simulink model "modelo_LTI_equivalente_dinamica_residual"  (R2020a)
settings: Solver=VariableStepAuto  StartTime=0.0  StopTime=10.0  RelTol=1e-3
model workspace: external: MATLAB File D:\Ferran\Facultad\UNCuyo\Meca\Automática y Máquinas Eléctricas\Proyecto final\matlab2\parametros_y_especs\parametros_y_especif.m (data not in the file)
undefined symbols (not defined in the file): beq, Cts, Jeq, lambda_m, Ld, Lq, magnitude, Pp, r, Rs, Rts_amb
settings Model: Creator=Ferran  LastModifiedBy=Ferran

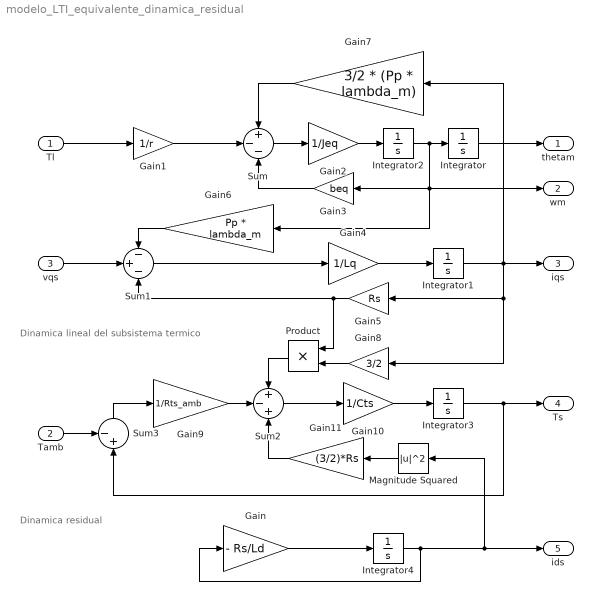
== system modelo_LTI_equivalente_dinamica_residual ==
  note: Dinamica residual
  note: Dinamica lineal del
      |  subsistema termico
  Tl : Inport
  Tamb : Inport  Port=2
  vqs : Inport  Port=3
  Gain : Gain  Gain=- Rs/Ld
  Gain1 : Gain  Gain=1/r
  Gain10 : Gain  Gain=1/Cts
  Gain11 : Gain  Gain=(3/2)*Rs
  Gain2 : Gain  Gain=1/Jeq
  Gain3 : Gain  Gain=beq
  Gain4 : Gain  Gain=1/Lq
  Gain5 : Gain  Gain=Rs
  Gain6 : Gain  Gain=Pp * lambda_m
  Gain7 : Gain  Gain=3/2 * (Pp * lambda_m)
  Gain8 : Gain  Gain=3/2
  Gain9 : Gain  Gain=1/Rts_amb
  Integrator{,1..4} (5 alike) : Integrator
  Magnitude Squared : Math  Operator=magnitude^2  SaturateOnIntegerOverflow=on
  Product : Product
  Sum : Sum  Inputs=+--
  Sum1 : Sum  Inputs=-+-
  Sum2 : Sum  Inputs=+-+
  Sum3 : Sum  Inputs=-+|
  thetam : Outport
  wm : Outport  Port=2
  iqs : Outport  Port=3
  Ts : Outport  Port=4
  ids : Outport  Port=5
  wires:
  Integrator/1 -> thetam/1
  Integrator2/1 -> Integrator/1, Gain6/1, wm/1, Gain3/1
  Gain2/1 -> Integrator2/1
  Tl/1 -> Gain1/1
  Gain1/1 -> Sum/2
  Gain3/1 -> Sum/3
  Sum/1 -> Gain2/1
  Sum1/1 -> Gain4/1
  Gain4/1 -> Integrator1/1
  Integrator1/1 -> Gain8/1, Gain5/1, Gain7/1, iqs/1
  Gain5/1 -> Product/1, Sum1/3
  vqs/1 -> Sum1/2
  Gain6/1 -> Sum1/1
  Gain7/1 -> Sum/1
  Gain8/1 -> Product/2
  Product/1 -> Sum2/1
  Tamb/1 -> Sum3/1
  Sum3/1 -> Gain9/1
  Gain9/1 -> Sum2/2
  Sum2/1 -> Gain10/1
  Gain10/1 -> Integrator3/1
  Integrator3/1 -> Sum3/2, Ts/1
  Gain/1 -> Integrator4/1
  Integrator4/1 -> Magnitude Squared/1, ids/1, Gain/1
  Magnitude Squared/1 -> Gain11/1
  Gain11/1 -> Sum2/3
